simulink model "spring_mass_model_01"  (R2014a)
settings: Solver=FixedStepDiscrete  StartTime=0.0  StopTime=inf  FixedStep=sample_time  RelTol=1e-3
values from neighbouring files (symbols this model uses):
  g = g_real    (= 9.803)    [max_motor_torques.m]
  l0_leg = 0.97    [max_motor_torques.m]
  l0_virtual = sqrt(d^2+l0_leg^2-2*d*l0_leg*cos(phi0))    [max_motor_torques.m]
undefined symbols (not defined in the file or in its folder): alpha_apex, alpha_max, alpha_min, boom_mount_angle, c_energy, contact_threshold, control_start_time, d_y_boom_com_offset, d_y_boom_hip_offset, d_y_com, d_y_mount_to_com, desired_torso_angle, DiscIntNeverNeededParam, dt_thrust, dx_avg_desired, extra_leg_damping, F_thrust, fcut_contact, ff_energy_l, ff_energy_r, g_reduced, h_boom, i_limit_lateral, i_robot, initial_com_height, initial_dt, initial_dx, j_leg, j_rotor, j_segments, k0_virtual, k_placement, k_sea, kd_flight, kd_lateral, kd_leg_angle, kd_motor, kd_raibert, kd_torso, ki_lateral, kp_flight_max, kp_flight_min, kp_lateral, kp_leg_angle, kp_motor, kp_raibert, kp_torso, l0_max_angle_error, l0_min_angle_error, l0_min_flight_time, l_boom, l_boom_projected, l_max, l_min, l_retract_escape, l_retract_swing, l_seg, lambda1, lambda2, lateral_offset ... (+33)
libraries: simulink x22, simulink_extras x2
(part 3 of 3)

== system spring_mass_model_01/Control/Behavior Control/Primary Leg Behavior/SMM 01/Primary Swing Phase/Leg Trajectory Generator (Level Ground)/Alpha Target Law l0 = 1.037112 m k = 23000 N//m target height = 1.137112 m target speed = 0.5 m//s m = 60.4120 kg g = 5.9004 m//s^2 E = 412.882588 J ==
  note: Angle of Attack Control Law From Poincare Map Method
  tFall [s] : Inport
  Alpha Target Polynomials : Subsystem
  AlphaRef1 : Constant  Value=[(90+20)*pi/180 0 0]
  Compare To Constant1 : simulink/Logic and Bit Operations/Compare To Constant  relop=<  const=0.19512514  OutDataTypeStr=boolean  ZeroCross=off
  Demux : Demux  Outputs=3
  Ignore Negatives : Fcn  Expr=(u >= 0)*u
  Mux : Mux  Inputs=3
  Switch : Switch  Criteria=u2 ~= 0
  AlphaRef(t) [rad] : Outport
  dAlphaRef(t) [rad/s] : Outport  Port=2
  ddAlphaRef(t) [rad/s^2] : Outport  Port=3
  wires:
  AlphaRef1/1 -> Switch/3
  Demux/3 -> ddAlphaRef(t) [rad/s^2]/1
  Demux/2 -> dAlphaRef(t) [rad/s]/1
  Demux/1 -> AlphaRef(t) [rad]/1
  Switch/1 -> Demux/1
  tFall [s]/1 -> Ignore Negatives/1, Compare To Constant1/1
  Compare To Constant1/1 -> Switch/2
  Alpha Target Polynomials/2(dAlphaRef(t)) -> Mux/2
  Alpha Target Polynomials/3(ddAlphaRef(t)) -> Mux/3
  Alpha Target Polynomials/1(AlphaRef(t)) -> Mux/1
  Mux/1 -> Switch/1
  Ignore Negatives/1 -> Alpha Target Polynomials/1(tFall)

== system spring_mass_model_01/Control/Behavior Control/Primary Leg Behavior/SMM 01/Primary Swing Phase/Leg Trajectory Generator (Level Ground)/Signal During Escape ==
  time : Inport
  Enable : EnablePort
  time to apex [s] : Outport
  wires:
  time/1 -> time to apex [s]/1

== system spring_mass_model_01/Control/Behavior Control/Primary Leg Behavior/SMM 01/Primary Swing Phase/Leg Trajectory Generator (Normal)/Alpha Target Law l0 = 1.037112 m k = 8820 N//m target height = 1.057112 m target speed = 1.0 m//s m = 60.4120 kg g = 5.900428 m//s^2 E = 444.778054 J ==
  note: Angle of Attack Control Law From Poincare Map Method
  tFall [s] : Inport
  Alpha Target Polynomials : Subsystem
  AlphaRef1 : Constant  Value=[(90+20)*pi/180 0 0]
  Compare To Constant1 : simulink/Logic and Bit Operations/Compare To Constant  relop=<  const=0.33124891  OutDataTypeStr=boolean  ZeroCross=off
  Demux : Demux  Outputs=3
  Ignore Negatives : Fcn  Expr=(u >= 0)*u
  Mux : Mux  Inputs=3
  Switch : Switch  Criteria=u2 ~= 0
  AlphaRef(t) [rad] : Outport
  dAlphaRef(t) [rad/s] : Outport  Port=2
  ddAlphaRef(t) [rad/s^2] : Outport  Port=3
  wires:
  Ignore Negatives/1 -> Alpha Target Polynomials/1(tFall)
  Mux/1 -> Switch/1
  Alpha Target Polynomials/3(ddAlphaRef(t)) -> Mux/3
  Alpha Target Polynomials/2(dAlphaRef(t)) -> Mux/2
  Compare To Constant1/1 -> Switch/2
  tFall [s]/1 -> Compare To Constant1/1, Ignore Negatives/1
  Switch/1 -> Demux/1
  Demux/1 -> AlphaRef(t) [rad]/1
  Demux/2 -> dAlphaRef(t) [rad/s]/1
  Demux/3 -> ddAlphaRef(t) [rad/s^2]/1
  AlphaRef1/1 -> Switch/3
  Alpha Target Polynomials/1(AlphaRef(t)) -> Mux/1

== system spring_mass_model_01/Control/Behavior Control/Primary Leg Behavior/SMM 01/Primary Stance Phase/Virtual Leg Force and Swing Leg Retraction/Hold Initial/Subsystem ==
  in : Inport
  Enable : EnablePort
  out : Outport  InitialOutput=[l0_virtual]
  wires:
  in/1 -> out/1

== system spring_mass_model_01/Control/Behavior Control/Primary Leg Behavior/SMM 01/Primary Stance Phase/Virtual Leg Force and Swing Leg Retraction/Touch Down Trigger/Timer ==
  Enable : EnablePort  StatesWhenEnabling=reset  ShowOutputPort=on
  Constant : Constant
  Discrete-Time Integrator : DiscreteIntegrator  IntegratorMethod=Accumulation: Forward Euler  gainval=sample_time  ExternalReset=rising  SampleTime=sample_time  ICPrevOutput=DiscIntNeverNeededParam  ICPrevScaledInput=DiscIntNeverNeededParam
  timer [s] : Outport  InitialOutput=[0]
  wires:
  Constant/1 -> Discrete-Time Integrator/1
  Enable/1 -> Discrete-Time Integrator/2
  Discrete-Time Integrator/1 -> timer [s]/1

== system spring_mass_model_01/Control/Behavior Control/Primary Leg Behavior/SMM 01/Primary Swing Phase/Leg Trajectory Generator (Level Ground)/Alpha Target Law l0 = 1.037112 m k = 23000 N//m target height = 1.137112 m target speed = 0.5 m//s m = 60.4120 kg g = 5.9004 m//s^2 E = 412.882588 J/Alpha Target Polynomials ==
  tFall : Inport
  AlphaRef(t) Control Law : Fcn  Expr=1.0339*u^3 + 6.848*u^2 + 3.5731*u + alpha_apex
  acceleration of AlphaRef(t) Control Law : Fcn  Expr=2*3*1.0339*u + 2*6.848
  velocity of AlphaRef(t) Control Law : Fcn  Expr=3*1.0339*u^2 + 2*6.848*u + 3.5731
  AlphaRef(t) : Outport  OutputWhenDisabled=reset  InitialOutput=0
      settings: AttributesFormatString=When disabled: %<OutputWhenDisabled>\nDisabled Output: %<InitialOutput>
  dAlphaRef(t) : Outport  Port=2  OutputWhenDisabled=reset  InitialOutput=0
      settings: AttributesFormatString=When disbaled: %<OutputWhenDisabled>\nDisabled output: %<InitialOutput>
  ddAlphaRef(t) : Outport  Port=3  OutputWhenDisabled=reset  InitialOutput=0
      settings: AttributesFormatString=When disabled: %<OutputWhenDisabled>\nDisabled output: %<InitialOutput>
  wires:
  acceleration of AlphaRef(t) Control Law/1 -> ddAlphaRef(t)/1
  velocity of AlphaRef(t) Control Law/1 -> dAlphaRef(t)/1
  AlphaRef(t) Control Law/1 -> AlphaRef(t)/1
  tFall/1 -> acceleration of AlphaRef(t) Control Law/1, velocity of AlphaRef(t) Control Law/1, AlphaRef(t) Control Law/1

== system spring_mass_model_01/Control/Behavior Control/Primary Leg Behavior/SMM 01/Primary Swing Phase/Leg Trajectory Generator (Normal)/Alpha Target Law l0 = 1.037112 m k = 8820 N//m target height = 1.057112 m target speed = 1.0 m//s m = 60.4120 kg g = 5.900428 m//s^2 E = 444.778054 J/Alpha Target Polynomials ==
  tFall : Inport
  AlphaRef(t) Control Law : Fcn  Expr=12.835*u^3 - 2.9736*u^2 + 1.9343*u + alpha_apex
  acceleration of AlphaRef(t) Control Law : Fcn  Expr=2*3*12.835*u - 2*2.9736
  velocity of AlphaRef(t) Control Law : Fcn  Expr=3*12.835*u^2 - 2*2.9736*u + 1.9343
  AlphaRef(t) : Outport  OutputWhenDisabled=reset  InitialOutput=0
      settings: AttributesFormatString=When disabled: %<OutputWhenDisabled>\nDisabled Output: %<InitialOutput>
  dAlphaRef(t) : Outport  Port=2  OutputWhenDisabled=reset  InitialOutput=0
      settings: AttributesFormatString=When disbaled: %<OutputWhenDisabled>\nDisabled output: %<InitialOutput>
  ddAlphaRef(t) : Outport  Port=3  OutputWhenDisabled=reset  InitialOutput=0
      settings: AttributesFormatString=When disabled: %<OutputWhenDisabled>\nDisabled output: %<InitialOutput>
  wires:
  tFall/1 -> AlphaRef(t) Control Law/1, velocity of AlphaRef(t) Control Law/1, acceleration of AlphaRef(t) Control Law/1
  AlphaRef(t) Control Law/1 -> AlphaRef(t)/1
  velocity of AlphaRef(t) Control Law/1 -> dAlphaRef(t)/1
  acceleration of AlphaRef(t) Control Law/1 -> ddAlphaRef(t)/1

== stateflow chart spring_mass_model_01/Control/Behavior Control/Primary Leg Behavior/Raibert  Hopper State Machine ==
  state Loading
    entry: placement = 0;
    entry: posture = 0;
    entry: thrust = 0;
    entry: flight = 0;
    entry: escape = 0;
  state Compression
    entry: placement = 0;
    entry: posture = 1;
    entry: thrust = 0;
    entry: flight = 0;
    entry: escape = 0;
  state Thrust
    entry: placement = 0;
    entry: posture = 1;
    entry: thrust = 1;
    entry: flight = 0;
    entry: escape = 0;
  state Unloading
    entry: placement = 0;
    entry: posture = 0;
    entry: thrust = 1;
    entry: flight = 0;
    entry: escape = 0;
  state Escape
    entry: placement = 0;
    entry: posture = 0;
    entry: thrust = 0;
    entry: flight = 1;
    entry: escape = 1;
  state Flight
    entry: placement = 1;
    entry: posture = 0;
    entry: thrust = 0;
    entry: flight = 1;
    entry: escape = 0;
  (junction 91) -> Loading
  Loading -> (junction 130) [order 2] : [Fy < contact_threshold]
  (junction 93) -> (junction 91)
  (junction 130) -> (junction 128)
  Loading -> Compression [order 1] : [Fy > loaded_threshold]
  (junction 115) -> Compression
  (junction 118) -> (junction 115)
  Compression -> Thrust : [dl >= 0 && dl_prev < 0]
  Thrust -> Unloading [order 1] : [Fy < loaded_threshold]
  Thrust -> (junction 102) [order 2] : [l > l_max]
  (junction 102) -> (junction 100)
  (junction 122) -> (junction 118)
  Unloading -> Escape [order 1] : [Fy < contact_threshold || l > l_max]
  Unloading -> (junction 122) [order 2] : [Fy > loaded_threshold]
  Escape -> Flight : after(t_flight,sec)
  (junction 100) -> Escape
  (default) -> Flight
  Flight -> (junction 93) : [Fy > contact_threshold]
  (junction 128) -> Flight
  data: flight output; escape output; thrust output; posture output; l input; dl input; dl_prev input; Fy input; t_flight parameter; placement output; l_max parameter; contact_threshold parameter; loaded_threshold parameter

== matlab function spring_mass_model_01/Control/Behavior Control/Primary Leg Behavior/SMM 01/Primary Swing Phase/Leg Trajectory Generator (Normal)/Avoid Virtual Leg Length Limits ==
  data: l_leg_desired input; dl_leg_desired input; ddl_leg_desired input; l_leg_cmd output double; dl_leg_cmd output double; ddl_leg_cmd output double; min_leg_length parameter; max_leg_length parameter
%% Avoid virtual leg length limits by ensuring we don't command position/velocities/accelerations that would hit them.
function [l_leg_cmd, dl_leg_cmd, ddl_leg_cmd] = AvoidVirtualLengthLimits(l_leg_desired, dl_leg_desired, ddl_leg_desired, min_leg_length, max_leg_length)
    [l_leg_cmd, dl_leg_cmd, ddl_leg_cmd] = AvoidVirtualLengthLimits(l_leg_desired, dl_leg_desired, ddl_leg_desired, min_leg_length, max_leg_length);
end

== matlab function spring_mass_model_01/Control/Behavior Control/Torque Distribution Right/Motor Torque Saturation Optimization ==
  data: x1s input; t1 output; x2s input; lambda1 parameter; lambda2 parameter; LEG_MTR_MAX_TORQUE parameter; t2 output
% Optimal leg motor torque distribution
function [t1, t2] = distribute_torque(x1s, x2s, lambda1, lambda2, LEG_MTR_MAX_TORQUE)

s = LEG_MTR_MAX_TORQUE;

% possible solutions
x1 = [                                                      x1s;
                                                            0;
                                                            s;
                                                            0;
                                                           -s;
  (lambda2*s + lambda1*x1s - lambda2*x2s)/(lambda1 + lambda2);
  (lambda1*x1s - lambda2*s + lambda2*x2s)/(lambda1 + lambda2);
  (lambda2*s + lambda1*x1s + lambda2*x2s)/(lambda1 + lambda2);
 -(lambda2*s - lambda1*x1s + lambda2*x2s)/(lambda1 + lambda2)];
 
x2 = [                                                      x2s;
                                                            s;
                                                            0;
                                                           -s;
                                                            0;
  (lambda1*s - lambda1*x1s + lambda2*x2s)/(lambda1 + lambda2);
  (lambda1*s + lambda1*x1s + lambda2*x2s)/(lambda1 + lambda2);
  (lambda1*x1s - lambda1*s + lambda2*x2s)/(lambda1 + lambda2);
 -(lambda1*s + lambda1*x1s - lambda2*x2s)/(lambda1 + lambda2)];

% test constraints
c1 = s - x1 - x2 >= 0;
c2 = s + x1 + x2 >= 0;
c3 = s - x1 + x2 >= 0;
c4 = s + x1 - x2 >= 0;
constraints = c1 & c2 & c3 & c4;

% objective function to maximize
f = -lambda1*(x1-x1s).^2-lambda2*(x2-x2s).^2;
satisfied = find(constraints);
[~,I] = max(f(satisfied));

t1 = x1(satisfied(I));
t2 = x2(satisfied(I));

== matlab function spring_mass_model_01/Control/Behavior Control/Primary Leg Behavior/Raibert Hopping/Virtual Leg Force and Swing Leg Retraction/Virtual Spring Force ==
  data: gamma input; dgamma input; gamma_tgt input; dgamma_tgt input; flight input; escape input; k_virtual input; l_spring input; F_virtual output; dl_spring input; l0_leg parameter; l_retract_escape parameter; l_retract_swing parameter; l_min parameter; l0_max_angle_error parameter; l0_min_angle_error parameter; kd_flight parameter; kp_flight_min parameter; kp_flight_max parameter; extra_leg_damping parameter; kd_raibert parameter
function F_virtual  = fcn(gamma, dgamma, gamma_tgt, dgamma_tgt, flight, escape, k_virtual, l_spring, dl_spring, ...
                          l0_leg, l_retract_escape, l_retract_swing, l_min,...
                          l0_max_angle_error, l0_min_angle_error,...
                          kd_flight, kp_flight_min, kp_flight_max, extra_leg_damping,...
                          kd_raibert)
                          
  if flight == 1
    %% Flight

    % modify length during swing
    l_target = l0_leg;
    if escape == 1
        l_target = l_retract_escape;
    else
        gamma_error = abs(gamma_tgt - gamma);
        slope = (l_retract_swing - l0_leg)/(l0_max_angle_error - l0_min_angle_error);
        l_target = l0_leg - slope*(l0_min_angle_error - gamma_error);
        l_target = min(max(l_target, l_retract_swing), l0_leg);
    end
    
    % compute leg force
    delta_l = l_target - l_spring;
    delta_dl = 0 - dl_spring;
    kp_flight = l_spring*-(kp_flight_max - kp_flight_min)/(l0_leg - l_min)+((kp_flight_max - kp_flight_min)/(l0_leg - l_min)*l0_leg+kp_flight_min);
    kp_flight = min(max(kp_flight, kp_flight_min), kp_flight_max);
    kd_flight = exp(-abs(1-l_spring/l0_leg)^0.8)*kd_flight;
    if l_spring > l0_leg
        kd_flight = kd_flight + extra_leg_damping;
    end
    F_virtual = kp_flight*delta_l + kd_flight*delta_dl;
    
  else  
    %% Stance
    l_target = l0_leg;
    %l_target = min(max(l_virtual_initial, l0_virtual_min),l0_virtual);
    delta_l = l_target - l_spring;
    delta_dl = 0 - dl_spring;
    F_virtual = max(0,k_virtual*delta_l + kd_raibert*delta_dl);
  end


end

== matlab function spring_mass_model_01/Control/Behavior Control/Secondary Leg Behavior/Avoid Hitting Mechanical Limits ==
  data: back_cmd output double; front_cmd output double; dback_cmd output double; dfront_cmd output double; ddback_cmd output double; ddfront_cmd output double; back_desired input; dback_desired input; ddback_desired input; front_desired input; dfront_desired input; ddfront_desired input; min_front_bar_angle parameter; max_front_bar_angle parameter; min_back_bar_angle parameter; max_back_bar_angle parameter
%% Avoid joint limits by ensuring we don't command velocities/accelerations that would push us into them when we are close to them.
function [back_cmd, front_cmd, dback_cmd, dfront_cmd, ddback_cmd, ddfront_cmd] ...
    = AvoidFourbarLimits(back_desired,dback_desired, ddback_desired, ...
          front_desired, dfront_desired, ddfront_desired, ...
          min_front_bar_angle, max_front_bar_angle, min_back_bar_angle, max_back_bar_angle)
    [back_cmd, front_cmd, dback_cmd, dfront_cmd, ddback_cmd, ddfront_cmd] = AvoidFourbarLimits(back_desired,dback_desired, ddback_desired, front_desired, dfront_desired, ddfront_desired, min_front_bar_angle, max_front_bar_angle, min_back_bar_angle, max_back_bar_angle);
end

== matlab function spring_mass_model_01/Control/Behavior Control/Velocity Estimation/dx_and_dy_from_yaw_and_roll ==
  data: qRoll input; dqRoll input; dx output; dqYaw input; dqPitch input; l_boom parameter; l_boom_projected parameter; h_boom parameter; boom_mount_angle parameter; d_y_boom_com_offset parameter; d_y_boom_hip_offset parameter; dy output; d_y_mount_to_com parameter; y_com output; y_hip output
function [dx, dy, y_com, y_hip] = fcn(qRoll, dqRoll, dqYaw, dqPitch, ...
                        l_boom, l_boom_projected, h_boom, boom_mount_angle, ...
                        d_y_boom_com_offset, d_y_boom_hip_offset, d_y_mount_to_com)
    % dx
    x_boom = l_boom * cos(qRoll);
    x_mount_to_center = d_y_mount_to_com * sin(qRoll-boom_mount_angle);
    dx = dqYaw * (x_boom + x_mount_to_center) - dqPitch * d_y_mount_to_com;
    
    % dy
    dy    = dqRoll * l_boom_projected * cos(qRoll)  +  d_y_boom_com_offset * dqRoll * sin(qRoll-boom_mount_angle);
    
    % y (COM and hip point)
    y_com = h_boom + l_boom_projected * sin(qRoll)  -  d_y_boom_com_offset * cos(qRoll-boom_mount_angle); 
    y_hip = h_boom + l_boom_projected * sin(qRoll)  -  d_y_boom_hip_offset * cos(qRoll-boom_mount_angle); 
end

== matlab function spring_mass_model_01/Control/Behavior Control/Torque Distribution Left/Motor Torque Saturation Optimization ==
  data: x1s input; t1 output; x2s input; lambda1 parameter; lambda2 parameter; LEG_MTR_MAX_TORQUE parameter; t2 output
% Optimal leg motor torque distribution
function [t1, t2] = distribute_torque(x1s, x2s, lambda1, lambda2, LEG_MTR_MAX_TORQUE)

s = LEG_MTR_MAX_TORQUE;

% possible solutions
x1 = [                                                      x1s;
                                                            0;
                                                            s;
                                                            0;
                                                           -s;
  (lambda2*s + lambda1*x1s - lambda2*x2s)/(lambda1 + lambda2);
  (lambda1*x1s - lambda2*s + lambda2*x2s)/(lambda1 + lambda2);
  (lambda2*s + lambda1*x1s + lambda2*x2s)/(lambda1 + lambda2);
 -(lambda2*s - lambda1*x1s + lambda2*x2s)/(lambda1 + lambda2)];
 
x2 = [                                                      x2s;
                                                            s;
                                                            0;
                                                           -s;
                                                            0;
  (lambda1*s - lambda1*x1s + lambda2*x2s)/(lambda1 + lambda2);
  (lambda1*s + lambda1*x1s + lambda2*x2s)/(lambda1 + lambda2);
  (lambda1*x1s - lambda1*s + lambda2*x2s)/(lambda1 + lambda2);
 -(lambda1*s + lambda1*x1s - lambda2*x2s)/(lambda1 + lambda2)];

% test constraints
c1 = s - x1 - x2 >= 0;
c2 = s + x1 + x2 >= 0;
c3 = s - x1 + x2 >= 0;
c4 = s + x1 - x2 >= 0;
constraints = c1 & c2 & c3 & c4;

% objective function to maximize
f = -lambda1*(x1-x1s).^2-lambda2*(x2-x2s).^2;
satisfied = find(constraints);
[~,I] = max(f(satisfied));

t1 = x1(satisfied(I));
t2 = x2(satisfied(I));

== matlab function spring_mass_model_01/Control/Behavior Control/Velocity Estimation/Takeoff Velocity/vertical_velocity ==
  data: y output; dx output; dy output double; l input; dl input; phi input; dphi input; qPitch input; dqPitch input; d_y_com parameter
function [y,dx,dy] = fcn(l, dl, phi, dphi, qPitch, dqPitch, d_y_com)

% y = -l*cos(theta+phi) + d*cos(theta)
% dy = -dl*cos(theta+phi) + l*(dtheta+dphi)*sin(theta+phi) - d*dtheta*sin(theta)
gamma = phi + qPitch;
dgamma = dphi + dqPitch;
d = d_y_com;

y = -l*cos(gamma) + d*cos(qPitch);
dy = -dl*cos(gamma) + l*dgamma*sin(gamma) - d*dqPitch*sin(qPitch);

% x = -l*sin(gamma) + d*sin(theta)
% dx = -dl*sin(gamma) - l*dgamma*cos(gamma) + d*dtheta*cos(theta)

dx = -dl*sin(gamma) - l*dgamma*cos(gamma) + d*dqPitch*cos(qPitch);

== matlab function spring_mass_model_01/Control/Behavior Control/Primary Leg Behavior/SMM 01/Primary Stance Phase/Virtual Leg Force and Swing Leg Retraction/target_GRF_inverse_dynamics ==
  data: z output; k_virtual input; l_virtual input; theta input; phi input; l_leg input; w input; tau_rotor_f input; tau_rotor_b input; d_y_com parameter; l0_virtual parameter; LEG_MTR_GEAR_RATIO parameter; g_reduced parameter; j_leg parameter; j_rotor parameter; i_robot parameter; m_total_real parameter; m_boom parameter; m_leg parameter; GRFx output; GRFy output; kp_torso parameter; kd_torso parameter; desired_torso_angle parameter; GRF_angle output; max_GRF_angle parameter
%% Inverse dynamics
% Inputs:  gamma, dgamma, theta, dtheta,  GRFx_des, GRFy_des
% Outputs: ddx,   ddy,    ddl,   ddgamma, ddtheta,  tau_sf,  tau_sb
function [z, GRFx, GRFy, GRF_angle]  = fcn(k_virtual, l_virtual, theta, phi, l_leg, w,...
                  tau_rotor_f, tau_rotor_b, ...
                  d_y_com, l0_virtual, LEG_MTR_GEAR_RATIO, g_reduced,...
                  j_leg, j_rotor, i_robot, ...
                  m_total_real, m_boom, m_leg, ...
                  kp_torso, kd_torso, desired_torso_angle, max_GRF_angle)

              
              
    % Parameters
    m      = m_total_real;    % mass of system + boom
    Il     = j_leg;             % inertia of leg
    Ir     = j_rotor;           % inertia of rotor
    It     = i_robot;           % inertia of system
    d      = d_y_com;             % distance from hip to system COM
    g1     = phi(1)+theta(1);   % global leg angle (after spring)
    dg1    = phi(2)+theta(2);
    th     = theta(1);          % global torso angle   
    dth    = theta(2);
    t_rf   = tau_rotor_f;       % torque applied at front rotor 
    t_rb   = tau_rotor_b;       % torque applied at back rotor
    N      = -LEG_MTR_GEAR_RATIO;
    l      = l_leg(1);          % leg length
    dl     = l_leg(2);
    lv     = l_virtual(1);      % virtual spring length
    dx     = -l*dg1*cos(g1)+dth*cos(th);
    dy     = l*dg1*sin(g1)-dth*sin(th);
    
    
    
    % Target GRFs
    delta_lv = l0_virtual -  lv;
    GRF = k_virtual*delta_lv* ...
                        [(d*sin(th)-l*sin(g1))/lv; ...
                         (d*cos(th)-l*cos(g1))/lv];
    GRF_angle = atan2(GRF(2),GRF(1));
                     
                     
                     
    % Trunk posture correction 
    F_reg = 1; % prevent division by zero
    ddth_desired = kp_torso*(desired_torso_angle - th) - kd_torso*dth; % PD law
    sine_ratio = It*ddth_desired / (lv*(norm(GRF) + F_reg));
    max_angle = 20*pi/180;
    sine_ratio = min(sin(max_angle), max(-sin(max_angle), sine_ratio));  % saturate rotation angle
    GRF_rotation = asin(sine_ratio);
    GRF_full_angle = GRF_rotation + GRF_angle; % saturate GRF angle
    if GRF_full_angle > (pi-max_GRF_angle)
        GRF_rotation = (pi-max_GRF_angle) - GRF_angle;
    elseif GRF_full_angle < max_GRF_angle
        GRF_rotation = max_GRF_angle - GRF_angle;  
    end
    R = [cos(GRF_rotation)  -sin(GRF_rotation); sin(GRF_rotation) cos(GRF_rotation)];
    GRF_target = R*GRF; % rotate GRF CCW
    GRFx = GRF_target(1);
    GRFy = GRF_target(2);
    GRF_angle = atan2(GRFy,GRFx);
    
    
    
    
    % Stance dynamics (P z = [h; -dJ*dq] + [J zeros(2,2)]^T F)
    %     J  = [1  0  sin(g1)     l*cos(g1)   -d*cos(th);
    %           0  1  cos(g1)    -l*sin(g1)    d*sin(th)];
    %       
    %     dJ = [0  0   dg1*cos(g1)    (-l*dg1*sin(g1)+dl*cos(g1))  d*dth*sin(th);
    %           0  0  -dg1*sin(g1)    (-1*dg1*cos(g1)-dl*sin(g1))  d*dth*cos(th)];
    % 
    %     dq  = [dx  dy  dl  dg1  dth ]';
    %       
    %     M = [m  0   0       0    0; 
    %          0  m   0       0    0;
    %          0  0   m_leg   0    0;   
    %          0  0   0       Il   0;  
    %          0  0   0       0    It];  
    %     
    %     h = [0; -m*g_reduced; 0; 0; (-t_rf-t_rb)];
    % 
    %     S = [ 0         0;
    %           0         0;
    %           1/w      -1/w;
    %           1         1;
    %          -(N-1)/N  -(N-1)/N];
    % 
    %     F = [GRFx GRFy]';
    %     
    %     P = [M              -S;       
    %          J               zeros(2,2)];
    
    % Solving for z:    
    %     ddq = [ddx ddy ddl ddg1 ddth]';
    %     z = [ddq; t_sf; t_sb];
    %     z = P\([h; -dJ*dq] + [J zeros(2,2)]'*F);
    
    z =  [GRFx/m;
         (GRFy - g_reduced*m)/m;
        -(Il*d*dg1^2*m*cos(g1 - th) - 2*GRFx*Il*d*sin(th) - 2*Il*d^2*dth^2*m - GRFy*d*l^2*m*cos(th) - GRFx*d*l^2*m*sin(th) - 2*GRFy*Il*d*cos(th) + 2*GRFy*It*N*l*cos(g1) + 2*GRFy*Il*N*d*cos(th) + 2*GRFx*It*N*l*sin(g1) + 2*GRFx*Il*N*d*sin(th) - It*N*dg1^2*l*m + GRFy*d*l^2*m*cos(2*g1 - th) + GRFx*d*l^2*m*sin(2*g1 - th) + 2*Il*d*g_reduced*m*cos(th) + Il*d*dg1^2*m*cos(g1 + th) + 2*Il*N*d^2*dth^2*m - It*N*dg1^2*l^2*m - 2*It*N*g_reduced*l*m*cos(g1) - 2*Il*N*d*g_reduced*m*cos(th) + It*N*dg1^2*l^2*m*cos(2*g1) - Il*N*d*dg1^2*m*cos(g1 + th) - Il*d*dg1^2*l*m*cos(g1 + th) + 4*Il*d*dg1*dl*m*sin(g1 - th) + GRFy*N*d^2*l*m*cos(g1) + GRFy*N*d*l^2*m*cos(th) + GRFx*N*d^2*l*m*sin(g1) + 2*N*d*l*m*t_rb*sin(g1 - th) + 2*N*d*l*m*t_rf*sin(g1 - th) + GRFx*N*d*l^2*m*sin(th) - Il*N*d*dg1^2*m*cos(g1 - th) - GRFy*N*d^2*l*m*cos(g1 - 2*th) + GRFx*N*d^2*l*m*sin(g1 - 2*th) + Il*d*dg1^2*l*m*cos(g1 - th) - It*N*dg1^2*l*m*cos(2*g1) - GRFy*N*d*l^2*m*cos(2*g1 - th) - GRFx*N*d*l^2*m*sin(2*g1 - th) + Il*N*d*dg1^2*l*m*cos(g1 + th) - 4*Il*N*d*dg1*dl*m*sin(g1 - th) - Il*N*d*dg1^2*l*m*cos(g1 - th) + 2*It*N*d*dth^2*l*m*cos(g1 - th))/(2*m*(It*N*l - Il*d*cos(g1 - th) + Il*N*d*cos(g1 - th)));
        -(2*GRFx*It*N*cos(g1) - 2*GRFy*It*N*sin(g1) + GRFx*N*d^2*m*cos(g1 - 2*th) + 4*It*N*dg1*dl*m + GRFy*N*d^2*m*sin(g1 - 2*th) + GRFx*d*l*m*cos(2*g1 - th) - GRFy*d*l*m*sin(2*g1 - th) + It*N*dg1^2*m*sin(2*g1) + 2*It*N*g_reduced*m*sin(g1) + GRFx*d*l*m*cos(th) - GRFy*d*l*m*sin(th) + GRFx*N*d^2*m*cos(g1) + 2*N*d*m*t_rb*cos(g1 - th) + 2*N*d*m*t_rf*cos(g1 - th) - GRFy*N*d^2*m*sin(g1) - GRFx*N*d*l*m*cos(th) + GRFy*N*d*l*m*sin(th) - GRFx*N*d*l*m*cos(2*g1 - th) - 2*It*N*d*dth^2*m*sin(g1 - th) + GRFy*N*d*l*m*sin(2*g1 - th) - It*N*dg1^2*l*m*sin(2*g1))/(2*m*(It*N*l - Il*d*cos(g1 - th) + Il*N*d*cos(g1 - th)));
        -(GRFx*Il*cos(g1) - GRFy*Il*sin(g1) - GRFx*Il*N*cos(g1) + (Il*dg1^2*m*sin(2*g1))/2 + GRFy*Il*N*sin(g1) + Il*g_reduced*m*sin(g1) + GRFx*l^2*m*cos(g1) - GRFy*l^2*m*sin(g1) + 2*Il*dg1*dl*m + N*l*m*t_rb + N*l*m*t_rf + GRFy*N*l^2*m*sin(g1) - 2*Il*N*dg1*dl*m - Il*d*dth^2*m*sin(g1 - th) - (Il*N*dg1^2*m*sin(2*g1))/2 - (Il*dg1^2*l*m*sin(2*g1))/2 - Il*N*g_reduced*m*sin(g1) - GRFx*N*l^2*m*cos(g1) + GRFx*N*d*l*m*cos(th) - GRFy*N*d*l*m*sin(th) + Il*N*d*dth^2*m*sin(g1 - th) + (Il*N*dg1^2*l*m*sin(2*g1))/2)/(m*(It*N*l - Il*d*cos(g1 - th) + Il*N*d*cos(g1 - th)));
        -(2*GRFx*Il*It*N*cos(g1) - 2*GRFy*Il*It*N*sin(g1) - GRFy*Il*d*m*w*cos(th) - 2*GRFy*Il*d*m_leg*w*cos(th) - GRFx*Il*d*m*w*sin(th) - 2*GRFx*Il*d*m_leg*w*sin(th) + GRFx*Il*N*d^2*m*cos(g1) + 2*Il*N*d*m*t_rb*cos(g1 - th) + 2*Il*N*d*m*t_rf*cos(g1 - th) + 2*GRFx*It*N*l^2*m*cos(g1) - GRFy*Il*N*d^2*m*sin(g1) - 2*GRFy*It*N*l^2*m*sin(g1) + GRFx*Il*N*d^2*m*cos(g1 - 2*th) + 4*Il*It*N*dg1*dl*m + GRFy*Il*N*d^2*m*sin(g1 - 2*th) - 2*Il*d^2*dth^2*m*m_leg*w - GRFy*Il*d*m*w*cos(2*g1 - th) - GRFx*Il*d*m*w*sin(2*g1 - th) + Il*It*N*dg1^2*m*sin(2*g1) + 2*Il*It*N*g_reduced*m*sin(g1) - GRFx*d*l^2*m*m_leg*w*sin(th) - Il*It*N*dg1^2*l*m*sin(2*g1) + Il*d*dg1^2*m*m_leg*w*cos(g1 - th) + 2*GRFy*It*N*l*m*w*cos(g1) + 2*GRFy*It*N*l*m_leg*w*cos(g1) + GRFy*Il*N*d*m*w*cos(th) + 2*GRFy*Il*N*d*m_leg*w*cos(th) + 2*GRFx*It*N*l*m*w*sin(g1) + 2*GRFx*It*N*l*m_leg*w*sin(g1) + GRFx*Il*N*d*m*w*sin(th) + 2*GRFx*Il*N*d*m_leg*w*sin(th) - It*N*dg1^2*l*m*m_leg*w + GRFy*d*l^2*m*m_leg*w*cos(2*g1 - th) + GRFx*d*l^2*m*m_leg*w*sin(2*g1 - th) + 2*Il*d*g_reduced*m*m_leg*w*cos(th) + Il*d*dg1^2*m*m_leg*w*cos(g1 + th) + 2*Il*N*d^2*dth^2*m*m_leg*w - It*N*dg1^2*l^2*m*m_leg*w - 2*Il*It*N*d*dth^2*m*sin(g1 - th) + GRFy*Il*N*d*m*w*cos(2*g1 - th) + GRFx*Il*N*d*m*w*sin(2*g1 - th) - GRFy*d*l^2*m*m_leg*w*cos(th) + It*N*dg1^2*l^2*m*m_leg*w*cos(2*g1) - Il*N*d*dg1^2*m*m_leg*w*cos(g1 + th) - Il*d*dg1^2*l*m*m_leg*w*cos(g1 + th) + 4*Il*d*dg1*dl*m*m_leg*w*sin(g1 - th) + GRFy*N*d^2*l*m*m_leg*w*cos(g1) + GRFy*N*d*l^2*m*m_leg*w*cos(th) + GRFx*N*d^2*l*m*m_leg*w*sin(g1) + 2*N*d*l*m*m_leg*t_rb*w*sin(g1 - th) + 2*N*d*l*m*m_leg*t_rf*w*sin(g1 - th) + GRFx*N*d*l^2*m*m_leg*w*sin(th) - Il*N*d*dg1^2*m*m_leg*w*cos(g1 - th) - GRFy*N*d^2*l*m*m_leg*w*cos(g1 - 2*th) + GRFx*N*d^2*l*m*m_leg*w*sin(g1 - 2*th) + Il*d*dg1^2*l*m*m_leg*w*cos(g1 - th) - It*N*dg1^2*l*m*m_leg*w*cos(2*g1) - GRFy*N*d*l^2*m*m_leg*w*cos(2*g1 - th) - GRFx*N*d*l^2*m*m_leg*w*sin(2*g1 - th) - 2*It*N*g_reduced*l*m*m_leg*w*cos(g1) - 2*Il*N*d*g_reduced*m*m_leg*w*cos(th) + Il*N*d*dg1^2*l*m*m_leg*w*cos(g1 + th) - 4*Il*N*d*dg1*dl*m*m_leg*w*sin(g1 - th) - Il*N*d*dg1^2*l*m*m_leg*w*cos(g1 - th) + 2*It*N*d*dth^2*l*m*m_leg*w*cos(g1 - th))/(4*m*(It*N*l - Il*d*cos(g1 - th) + Il*N*d*cos(g1 - th)));
         (2*GRFy*Il*It*N*sin(g1) - 2*GRFx*Il*It*N*cos(g1) - GRFy*Il*d*m*w*cos(th) - 2*GRFy*Il*d*m_leg*w*cos(th) - GRFx*Il*d*m*w*sin(th) - 2*GRFx*Il*d*m_leg*w*sin(th) - GRFx*Il*N*d^2*m*cos(g1) - 2*Il*N*d*m*t_rb*cos(g1 - th) - 2*Il*N*d*m*t_rf*cos(g1 - th) - 2*GRFx*It*N*l^2*m*cos(g1) + GRFy*Il*N*d^2*m*sin(g1) + 2*GRFy*It*N*l^2*m*sin(g1) - GRFx*Il*N*d^2*m*cos(g1 - 2*th) - 4*Il*It*N*dg1*dl*m - GRFy*Il*N*d^2*m*sin(g1 - 2*th) - 2*Il*d^2*dth^2*m*m_leg*w - GRFy*Il*d*m*w*cos(2*g1 - th) - GRFx*Il*d*m*w*sin(2*g1 - th) - Il*It*N*dg1^2*m*sin(2*g1) - 2*Il*It*N*g_reduced*m*sin(g1) - GRFx*d*l^2*m*m_leg*w*sin(th) + Il*It*N*dg1^2*l*m*sin(2*g1) + Il*d*dg1^2*m*m_leg*w*cos(g1 - th) + 2*GRFy*It*N*l*m*w*cos(g1) + 2*GRFy*It*N*l*m_leg*w*cos(g1) + GRFy*Il*N*d*m*w*cos(th) + 2*GRFy*Il*N*d*m_leg*w*cos(th) + 2*GRFx*It*N*l*m*w*sin(g1) + 2*GRFx*It*N*l*m_leg*w*sin(g1) + GRFx*Il*N*d*m*w*sin(th) + 2*GRFx*Il*N*d*m_leg*w*sin(th) - It*N*dg1^2*l*m*m_leg*w + GRFy*d*l^2*m*m_leg*w*cos(2*g1 - th) + GRFx*d*l^2*m*m_leg*w*sin(2*g1 - th) + 2*Il*d*g_reduced*m*m_leg*w*cos(th) + Il*d*dg1^2*m*m_leg*w*cos(g1 + th) + 2*Il*N*d^2*dth^2*m*m_leg*w - It*N*dg1^2*l^2*m*m_leg*w + 2*Il*It*N*d*dth^2*m*sin(g1 - th) + GRFy*Il*N*d*m*w*cos(2*g1 - th) + GRFx*Il*N*d*m*w*sin(2*g1 - th) - GRFy*d*l^2*m*m_leg*w*cos(th) + It*N*dg1^2*l^2*m*m_leg*w*cos(2*g1) - Il*N*d*dg1^2*m*m_leg*w*cos(g1 + th) - Il*d*dg1^2*l*m*m_leg*w*cos(g1 + th) + 4*Il*d*dg1*dl*m*m_leg*w*sin(g1 - th) + GRFy*N*d^2*l*m*m_leg*w*cos(g1) + GRFy*N*d*l^2*m*m_leg*w*cos(th) + GRFx*N*d^2*l*m*m_leg*w*sin(g1) + 2*N*d*l*m*m_leg*t_rb*w*sin(g1 - th) + 2*N*d*l*m*m_leg*t_rf*w*sin(g1 - th) + GRFx*N*d*l^2*m*m_leg*w*sin(th) - Il*N*d*dg1^2*m*m_leg*w*cos(g1 - th) - GRFy*N*d^2*l*m*m_leg*w*cos(g1 - 2*th) + GRFx*N*d^2*l*m*m_leg*w*sin(g1 - 2*th) + Il*d*dg1^2*l*m*m_leg*w*cos(g1 - th) - It*N*dg1^2*l*m*m_leg*w*cos(2*g1) - GRFy*N*d*l^2*m*m_leg*w*cos(2*g1 - th) - GRFx*N*d*l^2*m*m_leg*w*sin(2*g1 - th) - 2*It*N*g_reduced*l*m*m_leg*w*cos(g1) - 2*Il*N*d*g_reduced*m*m_leg*w*cos(th) + Il*N*d*dg1^2*l*m*m_leg*w*cos(g1 + th) - 4*Il*N*d*dg1*dl*m*m_leg*w*sin(g1 - th) - Il*N*d*dg1^2*l*m*m_leg*w*cos(g1 - th) + 2*It*N*d*dth^2*l*m*m_leg*w*cos(g1 - th))/(4*m*(It*N*l - Il*d*cos(g1 - th) + Il*N*d*cos(g1 - th)))];


end

== matlab function spring_mass_model_01/Control/Behavior Control/Primary Leg Behavior/SMM 01/Primary Swing Phase/Leg Trajectory Generator (Normal)/Alpha Target to Leg Length and Leg Angle ==
  data: alpha_v input; dalpha_v input; ddalpha_v input; theta input; dtheta input; l output; dl output; ddl output; phi output; d_y_com parameter; l0_virtual parameter; dphi output; ddphi output
function [l, dl, ddl, phi, dphi, ddphi] = fcn(alpha_v, dalpha_v, ddalpha_v, theta, dtheta, d_y_com, l0_virtual)
    [l, dl, ddl, phi, dphi, ddphi] = AlphaTargetToVirtualLeg2D(alpha_v, dalpha_v, ddalpha_v, theta, dtheta, 0, d_y_com, l0_virtual);
end

== matlab function spring_mass_model_01/Control/Behavior Control/Virtual Spring Calculator/Virtual Spring Calculations ==
  data: th input; alpha_v output; dth input; l input; dl input; phi input; dphi input; dalpha_v output; l_v output; dl_v output; d_y_com parameter
function [alpha_v, dalpha_v, l_v, dl_v] = fcn(th, dth, l, dl, phi, dphi, d_y_com)

gma = th + phi;
dgma = dth + dphi;
d = d_y_com;

xf  =  l*sin(gma) - d*sin(th);
dxf =  l*dgma*cos(gma) + dl*sin(gma) - d*dth*cos(th);
yf  = -l*cos(gma) + d*cos(th);
dyf =  l*dgma*sin(gma) - dl*cos(gma) - d*dth*sin(th);

alpha_v  = atan2(yf, xf);
dalpha_v = 1/(1+(yf/xf)^2) * (xf*dyf - yf*dxf)/xf^2;

l_v  = (d^2 + l^2 - 2*d*l*cos(phi))^0.5;
dl_v = (l*dl - d*dl*cos(phi) + d*l*dphi*sin(phi))/l_v;

end

== matlab function spring_mass_model_01/Control/Behavior Control/Primary Leg Behavior/SMM 01/Primary Swing Phase/Leg Trajectory Generator (Normal)/Retracted Leg Trajectory ==
  data: start input boolean; t_system input double; t_apex input double; l_apex input double; dl_apex input double; phi_apex input double; dphi_apex input double; l_measured input double; dl_measured input double; phi_measured input double; l output double; dl output double; ddl output double; phi output double; dphi output double; ddphi output double; dphi_measured input double
%% Generates a dynamically feasible trajectory for swinging the virtual leg between two points.
% Constrains to starting/ending positions and velocities.
% Minimizes torque squared
% May want to generate the trajectory in fourbar coordinates instead.
function [l, dl, ddl, phi, dphi, ddphi] = fcn(start, t_system, t_apex, l_apex, dl_apex, phi_apex, dphi_apex, l_measured, dl_measured, phi_measured, dphi_measured)

    persistent t_start l_start phi_start dl_start dphi_start;
    if isempty(t_start)
        t_start = t_system;
        l_start = l_measured;
        dl_start = dl_measured;
        phi_start = phi_measured;
        dphi_start = dphi_measured;
    end
    if start %|| (t_system - t_start) > 0.030
        t_start = t_system;
        l_start = l_measured;
        dl_start = dl_measured;
        phi_start = phi_measured;
        dphi_start = dphi_measured;
    end
    
    t = t_system - t_start;
    time_to_apex = t_apex - t_start;
    t = min(time_to_apex, t);

    % Virtual Leg Length
    [a0, a1, a2, a3] = ThirdOrderTrajectory(l_start, dl_start, l_apex, dl_apex, time_to_apex);
    l = a3*t^3 + a2*t^2 + a1*t + a0;
    dl = 3*a3*t^2 + 2*a2*t + a1;
    ddl = 6*a3*t + 2*a2;
    
    % Virtual Leg Angle
    [a0, a1, a2, a3] = ThirdOrderTrajectory(phi_start, dphi_start, phi_apex, dphi_apex, time_to_apex);
    phi = a3*t^3 + a2*t^2 + a1*t + a0;
    dphi = 3*a3*t^2 + 2*a2*t + a1;
    ddphi = 6*a3*t + 2*a2;

end

== matlab function spring_mass_model_01/Control/Behavior Control/Primary Leg Behavior/SMM 01/Primary Swing Phase/Virtual Leg to Four Bar ==
  data: l_leg input; dl_leg input; ddl_leg input; phi input; dphi input; ddphi input; back output; dback output; ddback output; front output; dfront output; ddfront output
function [back, dback, ddback, front, dfront, ddfront] = VirtualLegToFourBar(l_leg, dl_leg, ddl_leg, phi, dphi, ddphi)   
    [back, dback, ddback, front, dfront, ddfront] = VirtualLegToFourBar(l_leg, dl_leg, ddl_leg, phi, dphi, ddphi);
end

== matlab function spring_mass_model_01/Control/Behavior Control/Primary Leg Behavior/SMM 01/Primary Swing Phase/Leg Trajectory Generator (Normal)/Avoid Virtual Leg Length Limits1 ==
  data: l_leg_desired input; dl_leg_desired input; ddl_leg_desired input; l_leg_cmd output double; dl_leg_cmd output double; ddl_leg_cmd output double; min_leg_length parameter; max_leg_length parameter
%% Avoid virtual leg length limits by ensuring we don't command position/velocities/accelerations that would hit them.
function [l_leg_cmd, dl_leg_cmd, ddl_leg_cmd] = AvoidVirtualLengthLimits(l_leg_desired, dl_leg_desired, ddl_leg_desired, min_leg_length, max_leg_length)
    [l_leg_cmd, dl_leg_cmd, ddl_leg_cmd] = AvoidVirtualLengthLimits(l_leg_desired, dl_leg_desired, ddl_leg_desired, min_leg_length, max_leg_length);
end

== matlab function spring_mass_model_01/Control/Behavior Control/Secondary Leg Behavior/Virtual Leg Trajectory Towards Alpha Apex Target ==
  data: start input; t_system input; l_leg output; dl_leg output; ddl_leg output; phi output; dphi output; ddphi output; alpha_apex parameter; theta input; l_measured input; dl_measured input; phi_measured input; dphi_measured input; d_y_com parameter; l0_virtual parameter
%% Create a trajectory between starting position/velocity and some alpha
% The goal is to move the system towards the alpha target at apex.
function [l_leg, dl_leg, ddl_leg, phi, dphi, ddphi] = fcn(start, t_system, alpha_apex, theta, l_measured, dl_measured, phi_measured, dphi_measured, d_y_com, l0_virtual)
    % Should the target be less than apex position? midpoint?
    [l_apex, dl_apex, ~, phi_apex, dphi_apex, ~] = AlphaTargetToVirtualLeg2D(alpha_apex, 0, 0, theta, 0, 0, d_y_com, l0_virtual);
    
    % Force retraction when secondary leg
    l_apex = 0.8;
    dl_apex = 0;
    
    persistent t_start l_start phi_start dl_start dphi_start;
    if isempty(t_start)
        t_start = t_system;
        l_start = l_measured;
        dl_start = dl_measured;
        phi_start = phi_measured;
        dphi_start = dphi_measured;
    end
    if start %|| (t_system - t_start) > 0.030
        t_start = t_system;
        l_start = l_measured;
        dl_start = dl_measured;
        phi_start = phi_measured;
        dphi_start = dphi_measured;
    end
    

    time_to_takeoff = 0.350;  % Overestimate, How to approximate this?
    t = t_system - t_start;
    t = min(time_to_takeoff, t);
    
    % Virtual Leg Length
    [a0, a1, a2, a3] = ThirdOrderTrajectory(l_start, dl_start, l_apex, dl_apex, time_to_takeoff);
    l_leg = a3*t^3 + a2*t^2 + a1*t + a0;
    dl_leg = 3*a3*t^2 + 2*a2*t + a1;
    ddl_leg = 6*a3*t + 2*a2;
    
    % Virtual Leg Angle
    [a0, a1, a2, a3] = ThirdOrderTrajectory(phi_start, dphi_start, phi_apex, dphi_apex, time_to_takeoff);
    phi = a3*t^3 + a2*t^2 + a1*t + a0;
    dphi = 3*a3*t^2 + 2*a2*t + a1;
    ddphi = 6*a3*t + 2*a2;
end

== matlab function spring_mass_model_01/Control/Behavior Control/Secondary Leg Behavior/Virtual Leg to Four Bar ==
  data: l_leg input; dl_leg input; ddl_leg input; phi input; dphi input; ddphi input; back output; dback output; ddback output; front output; dfront output; ddfront output
function [back, dback, ddback, front, dfront, ddfront] = VirtualLegToFourBar(l_leg, dl_leg, ddl_leg, phi, dphi, ddphi)
    [back, dback, ddback, front, dfront, ddfront] = VirtualLegToFourBar(l_leg, dl_leg, ddl_leg, phi, dphi, ddphi);
end

== matlab function spring_mass_model_01/Control/Behavior Control/Primary Leg Behavior/SMM 01/Primary Swing Phase/Leg Trajectory Generator (Level Ground)/Alpha Target to Leg Length and Leg Angle ==
  data: alpha_v input; dalpha_v input; ddalpha_v input; theta input; dtheta input; l output; dl output; ddl output; phi output; d_y_com parameter; l0_virtual parameter; dphi output; ddphi output
function [l, dl, ddl, phi, dphi, ddphi] = fcn(alpha_v, dalpha_v, ddalpha_v, theta, dtheta, d_y_com, l0_virtual)
    [l, dl, ddl, phi, dphi, ddphi] = AlphaTargetToVirtualLeg2D(alpha_v, dalpha_v, ddalpha_v, theta, dtheta, 0, d_y_com, l0_virtual);
end

== matlab function spring_mass_model_01/Control/Behavior Control/Primary Leg Behavior/SMM 01/Primary Swing Phase/Leg Trajectory Generator (Level Ground)/Retracted Leg Trajectory ==
  data: start input; t_system input; t_apex input; l_apex input; dl_apex input; phi_apex input; dphi_apex input; l_measured input; dl_measured input; phi_measured input; l output; dl output; ddl output; phi output; dphi output; ddphi output; dphi_measured input
%% Generates a dynamically feasible trajectory for swinging the virtual leg between two points.
% Constrains to starting/ending positions and velocities.
% Minimizes torque squared
% May want to generate the trajectory in fourbar coordinates instead.
function [l, dl, ddl, phi, dphi, ddphi] = fcn(start, t_system, t_apex, l_apex, dl_apex, phi_apex, dphi_apex, l_measured, dl_measured, phi_measured, dphi_measured)

    persistent t_start l_start phi_start dl_start dphi_start;
    if isempty(t_start) || start
        t_start = t_system;
        l_start = l_measured;
        dl_start = dl_measured;
        phi_start = phi_measured;
        dphi_start = dphi_measured;
    end
    
    t = t_system - t_start;
    time_to_apex = 0.95*2*(t_apex - t_start);
    t = min(time_to_apex, t);

    % Virtual Leg Length
    [a0, a1, a2, a3] = ThirdOrderTrajectory(l_start, dl_start, l_apex, dl_apex, time_to_apex);
    l = a3*t^3 + a2*t^2 + a1*t + a0;
    dl = 3*a3*t^2 + 2*a2*t + a1;
    ddl = 6*a3*t + 2*a2;
    
    % Virtual Leg Angle
    [a0, a1, a2, a3] = ThirdOrderTrajectory(phi_start, dphi_start, phi_apex, dphi_apex, time_to_apex);
    phi = a3*t^3 + a2*t^2 + a1*t + a0;
    dphi = 3*a3*t^2 + 2*a2*t + a1;
    ddphi = 6*a3*t + 2*a2;

end

== matlab function spring_mass_model_01/Control/Behavior Control/Primary Leg Behavior/SMM 01/Primary Swing Phase/Avoid Hitting Mechanical Limits1 ==
  data: back_cmd output; front_cmd output; dback_cmd output; dfront_cmd output; ddback_cmd output; ddfront_cmd output; back_desired input; dback_desired input; ddback_desired input; front_desired input; dfront_desired input; ddfront_desired input; min_front_bar_angle parameter; max_front_bar_angle parameter; min_back_bar_angle parameter; max_back_bar_angle parameter
%% Avoid joint limits by ensuring we don't command velocities/accelerations that would push us into them when we are close to them.
function [back_cmd, front_cmd, dback_cmd, dfront_cmd, ddback_cmd, ddfront_cmd] ...
    = AvoidFourbarLimits(back_desired,dback_desired, ddback_desired, ...
          front_desired, dfront_desired, ddfront_desired, ...
          min_front_bar_angle, max_front_bar_angle, min_back_bar_angle, max_back_bar_angle)
    [back_cmd, front_cmd, dback_cmd, dfront_cmd, ddback_cmd, ddfront_cmd] = AvoidFourbarLimits(back_desired,dback_desired, ddback_desired, front_desired, dfront_desired, ddfront_desired, min_front_bar_angle, max_front_bar_angle, min_back_bar_angle, max_back_bar_angle);
end

== matlab function spring_mass_model_01/Control/Behavior Control/Primary Secondary Leg Swap/ToggleRightLeftLeg ==
  data: toggle input boolean; right_left output double; previous_right_left input double
function right_left = ToggleRightLeftLeg(toggle, previous_right_left)
    
    if toggle
        right_left = -previous_right_left + 1;
    else
        right_left = previous_right_left;
    end

end
